simulink model "dc_motor"  (R2021a)
settings: Solver=FixedStepAuto  StartTime=0.0  StopTime=20  FixedStep=0.01  RelTol=1e-3  EnableMultiTasking=on
libraries: adrc_toolbox_library x1, arduinomotorcarrierlib x1, mkrmotorcarrierlib x1
settings Model: SimulationMode=external  SILPILModeSetting=veronly  ExtModeTrigDuration=2  Creator=Krzysztof  LastModifiedBy=PC
settings SolverCC: AlgebraicLoopSolver=TrustRegion
settings DataIOCC: SaveFormat=StructureWithTime
settings OptimizationCC: EnhancedBackFolding=on  PassReuseOutputArgsThreshold=0  MaxStackSize=64  OptimizeBlockOrder=speed  DifferentSizesBufferReuse=on  OptimizationCustomize=off
settings DebuggingCC: ParameterTunabilityLossMsg=error  SFMachineParentedDataDiag=warning
settings HardwareCC: ProdBitPerPointer=32  ProdBitPerSizeT=32  ProdBitPerPtrDiffT=32  ProdLargestAtomicInteger=Long  ProdLargestAtomicFloat=Double  ProdWordSize=32  ProdLongLongMode=on  ProdHWDeviceType=ARM Compatible->ARM Cortex  UseEmbeddedCoderFeatures=off  UseSimulinkCoderFeatures=off
settings SFSimCC: MATLABDynamicMemAlloc=off
settings RTWCC: SystemTargetFile=ert.tlc  HardwareBoard=Arduino MKR WiFi 1010  TemplateMakefile=ert_default_tmf  Toolchain=Arduino ARM  BuildConfiguration=Faster Runs
settings CodeAppCC: ForceParamTrailComments=on  OperatorAnnotations=on  MangleLength=10
settings ERTTargetCC: ERTCustomFileBanners=off  SupportContinuousTime=on  SupportNonInlinedSFcns=on  RemoveResetFunc=off  SupportVariableSizeSignals=on  ModelStepFunctionPrototypeControlCompliant=off  ExtModeStaticAllocSize=8192

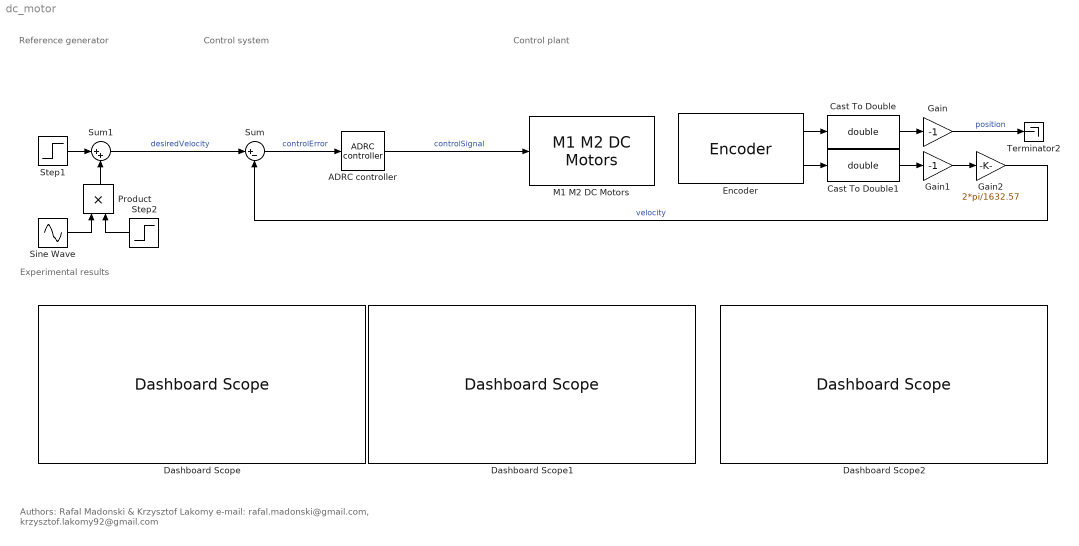
== system dc_motor ==
  note: Control system
  note: Control plant
  note: Reference
      | generator
  note: Experimental results
  note: Authors:  Rafal Madonski & Krzysztof Lakomy
      | e-mail: rafal.madonski@gmail.com, krzysztof.lakomy92@gmail.com
  ADRC controller : adrc_toolbox_library/ADRC controller  dynamicsOrder=2  controllerBandwidth=40  controllerBandwidthSource=Internal  observerBandwidth=90  observerBandwidthSource=Internal  inputGainParameter=600  inputGainSource=Internal  saturationEnabled=on  UpperLimit=100  LowerLimit=-100  antiPeakingEnabled=off  antiPeakingTime=0.2
      link override State feedback robust controller/Saturation: VariantControlMode=label  LabelModeActiveChoice=saturation_off
      settings: SourceProductName=ADRC toolbox
  Cast To Double : DataTypeConversion  OutDataTypeStr=double
  Cast To Double1 : DataTypeConversion  OutDataTypeStr=double
  Dashboard Scope : DashboardScope
  Dashboard Scope1 : DashboardScope
  Dashboard Scope2 : DashboardScope  Ymin=-0.1  Ymax=0.1
  Encoder : arduinomotorcarrierlib/Encoder  SlaveAddress=uint8( hex2dec( '66' ) )  blockPlatform=ARDUINO  Encoder=1  ShowSpeed=on  ResetOption=on  SampleTime=0.01
      settings: SourceProductBaseCode=ARDUINO
  Gain : Gain  Gain=-1  OutDataTypeStr=double
  Gain1 : Gain  Gain=-1  ParamDataTypeStr=double
  Gain2 : Gain  Gain=2*pi/1632.57
  M1 M2 DC Motors : mkrmotorcarrierlib/M1 M2 DC Motors  SlaveAddress=uint8( hex2dec( '66' ) )  blockPlatform=ARDUINO  MotorNumber=M1  MotorCarrierPWMFreq=100
      settings: SourceProductBaseCode=ARDUINO
  Product : Product
  Sine Wave : Sin  Amplitude=5  Frequency=6.28/4  SampleTime=0
  Step1 : Step  Time=3  After=15  SampleTime=0
  Step2 : Step  Time=3  SampleTime=0
  Sum : Sum  Inputs=|+-
  Sum1 : Sum  Inputs=|++
  Terminator2 : Terminator
  wires:
  Sum/1 -> ADRC controller/1  "controlError"
  ADRC controller/1 -> M1 M2 DC Motors/1  "controlSignal"
  Cast To Double1/1 -> Gain1/1
  Encoder/1 -> Cast To Double/1
  Encoder/2 -> Cast To Double1/1
  Cast To Double/1 -> Gain/1
  Gain/1 -> Terminator2/1  "position"
  Step1/1 -> Sum1/1
  Product/1 -> Sum1/2
  Sine Wave/1 -> Product/1
  Step2/1 -> Product/2
  Sum1/1 -> Sum/1  "desiredVelocity"
  Gain1/1 -> Gain2/1
  Gain2/1 -> Sum/2  "velocity"
